simulink model "bike_shock_sim"  (R2024b)
settings: Solver=VariableStepAuto  StartTime=0.0  StopTime=10.0  RelTol=1e-3
settings Model: Creator=alexa  LastModifiedBy=alexa

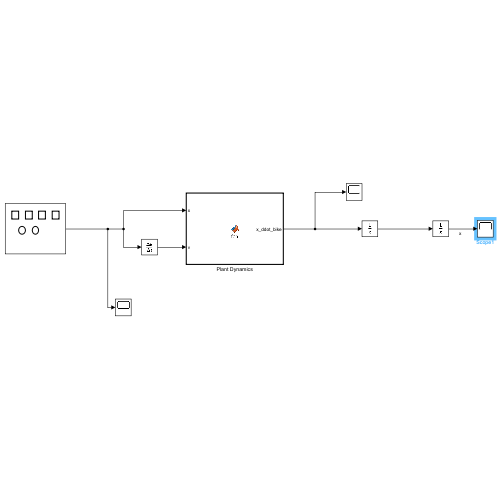
[thumbnail: Simulink's stored preview of the top-level diagram]
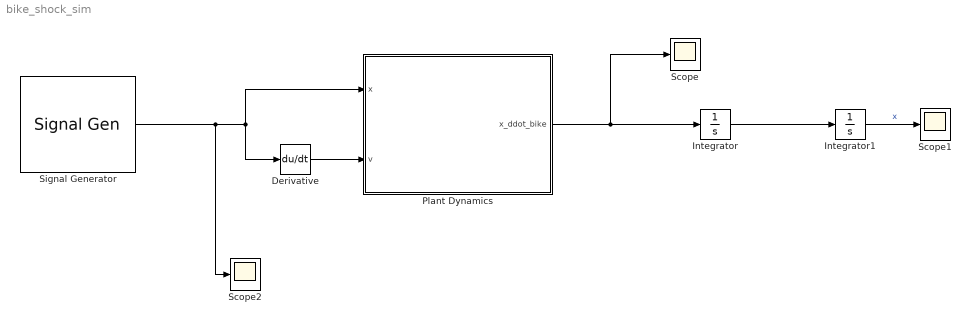
== system bike_shock_sim ==
  Derivative : Derivative
  Integrator : Integrator
  Integrator1 : Integrator
  Plant Dynamics : MATLAB Function  TreatAsAtomicUnit=on
  Scope : Scope
  Scope1 : Scope
  Scope2 : Scope
  Signal Generator : SignalGenerator  Units=rad/sec
  wires:
  Signal Generator/1 -> Scope2/1, Derivative/1, Plant Dynamics/1(x)
  Derivative/1 -> Plant Dynamics/2(v)
  Plant Dynamics/1(x_ddot_bike) -> Integrator/1, Scope/1
  Integrator/1 -> Integrator1/1
  Integrator1/1 -> Scope1/1  "x"

== matlab function bike_shock_sim/Plant Dynamics ==
  data: x input; x_ddot_bike output; v input
function x_ddot_bike = fcn(x, v)
%spring-damper in parallel

k = 1;
b = 0.1;
m_bike = 10;

F = -k*x-b*v;

x_ddot_bike = F/m_bike;
